simulink model "sf_bridge"  (Simulink 7.6)
settings: Solver=ode45  StartTime=0.0  StopTime=inf  RelTol=1e-3
libraries: sf_bidder x4, simulink x1
CloseFcn:
  | delete(findall(0, 'type', 'figure', 'tag', 'SF_BRIDGE'));
settings Model: Creator=The MathWorks Inc.  CovMetricSettings=dcmtr  ExtModeAutoUpdateStatusClock=off
settings DataIOCC: SignalLoggingName=sigsOut
settings OptimizationCC: InitFltsAndDblsToZero=on
settings DebuggingCC: SaveWithParameterizedLinksMsg=none  CheckExecutionContextPreStartOutputMsg=on  CheckExecutionContextRuntimeOutputMsg=on  SignalResolutionControl=TryResolveAllWithWarning  SolverPrmCheckMsg=none  MultiTaskDSMMsg=warning  MultiTaskCondExecSysMsg=none  StrictBusMsg=None
settings HardwareCC: TargetUnknown=on
settings SFSimCC: SFSimOverflowDetection=off  SimParseCustomCode=off
settings RTWCC: IncludeERTFirstTime=on
settings GRTTargetCC: TargetFcnLib=ansi_tfl_tmw.mat

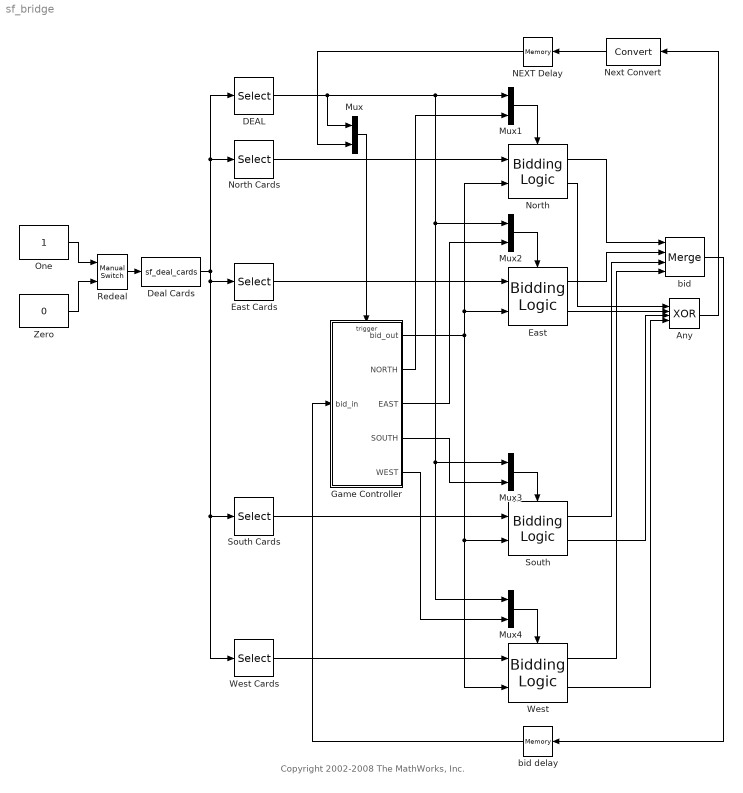
== system sf_bridge ==
  note: Copyright 2002-2008 The MathWorks, Inc.
  Any : Logic  Operator=XOR  Inputs=4  AllPortsSameDT=off
  DEAL : Selector  InputPortWidth=53  IndexOptions=Index vector (dialog)  Indices=[1]  OutputSizes=1
  Deal Cards : MATLABFcn  MATLABFcn=sf_deal_cards  OutputDimensions=53
  East : sf_bidder/Bidding Logic  SystemSampleTime=-1
  East Cards : Selector  InputPortWidth=53  IndexOptions=Index vector (dialog)  Indices=[15:27]  OutputSizes=1
  Game Controller : Stateflow chart  TreatAsAtomicUnit=on
  Mux{,1..4} (5 alike) : Mux  Inputs=2
  NEXT Delay : Memory
  Next Convert : DataTypeConversion  SaturateOnIntegerOverflow=on  RndMeth=Zero
  North : sf_bidder/Bidding Logic  SystemSampleTime=-1
  North Cards : Selector  InputPortWidth=53  IndexOptions=Index vector (dialog)  Indices=[2:14]  OutputSizes=1
  One : Constant
  Redeal : simulink/Signal Routing/Manual Switch  SystemSampleTime=-1  sw=0  action=0  varsize=off
  South : sf_bidder/Bidding Logic  SystemSampleTime=-1
  South Cards : Selector  InputPortWidth=53  IndexOptions=Index vector (dialog)  Indices=[28:40]  OutputSizes=1
  West : sf_bidder/Bidding Logic  SystemSampleTime=-1
  West Cards : Selector  InputPortWidth=53  IndexOptions=Index vector (dialog)  Indices=[41:53]  OutputSizes=1
  Zero : Constant  Value=0
  bid : Merge  Inputs=4
  bid delay : Memory
  wires:
  Deal Cards/1 -> DEAL/1, North Cards/1, West Cards/1, South Cards/1, East Cards/1
  DEAL/1 -> Mux/1, Mux1/1, Mux2/1, Mux4/1, Mux3/1
  bid/1 -> bid delay/1
  Any/1 -> Next Convert/1
  North Cards/1 -> North/1
  East Cards/1 -> East/1
  South Cards/1 -> South/1
  West Cards/1 -> West/1
  Game Controller/1(bid_out) -> South/2, West/2, North/2, East/2
  North/1 -> bid/1
  East/1 -> bid/2
  South/1 -> bid/3
  West/1 -> bid/4
  bid delay/1 -> Game Controller/1(bid_in)
  NEXT Delay/1 -> Mux/2
  Mux/1 -> Game Controller/Trigger
  North/2 -> Any/1
  West/2 -> Any/4
  East/2 -> Any/2
  South/2 -> Any/3
  Next Convert/1 -> NEXT Delay/1
  Mux1/1 -> North/Trigger
  Mux2/1 -> East/Trigger
  Mux3/1 -> South/Trigger
  Mux4/1 -> West/Trigger
  Game Controller/2(NORTH) -> Mux1/2
  Game Controller/3(EAST) -> Mux2/2
  Game Controller/4(SOUTH) -> Mux3/2
  Game Controller/5(WEST) -> Mux4/2
  Redeal/1 -> Deal Cards/1
  One/1 -> Redeal/1
  Zero/1 -> Redeal/2

== stateflow chart Game Controller ==
  state Bidder [parallel]
    settings: executionOrder=1
    state North
      NORTH;
    state East
      EAST;
    state South
      SOUTH;
    state West
      WEST;
    state Done
    Bidder -> (junction 21) [order 1] : BID
        | {process_bid();}
    Bidder.South -> Bidder.West : NEXT_BID
    Bidder.West -> Bidder.North : NEXT_BID
    Bidder.North -> Bidder.East : NEXT_BID
    Bidder.East -> Bidder.South : NEXT_BID
    (default) -> Done
    Done -> Bidder.North [order 2] : N_DEAL
    Done -> Bidder.East [order 1] : E_DEAL
    Done -> Bidder.South [order 4] : S_DEAL
    Done -> Bidder.West [order 3] : W_DEAL
    Bidder -> (junction 15) [order 3] : DEAL
        | {pass_count = 0;
        | bid_out = 0;}
    Bidder -> Done [order 2] : ALL_PASS
        | {ml.sf_bridge_state('all_pass');}
  state process_bid() [function]
    (junction 20) -> (junction 17) [order 1] : [bid_out]
        | {ALL_PASS;}
    (junction 20) -> (junction 24) [order 2] : {NEXT_BID;}
    (junction 19) -> (junction 23) [order 3] : {NEXT_BID;}
    (junction 16) -> (junction 19) [order 2] : {pass_count++;}
    (junction 16) -> (junction 18) [order 1] : [bid_in]
        | {pass_count = 0;
        | bid_out = bid_in;
        | NEXT_BID;}
    (junction 19) -> (junction 22) [order 1] : [pass_count == 4]
        | {ALL_PASS;}
    (default) -> (junction 16) : {ml.sf_bridge_state('bid', bid_in);}
    (junction 19) -> (junction 20) [order 2] : [pass_count == 3]
  state Dealer [parallel]
    settings: executionOrder=2
    state North
      ml.sf_bridge_state('deal', 'North');
      N_DEAL;
    state West
      ml.sf_bridge_state('deal', 'West');
      W_DEAL;
    state East
      ml.sf_bridge_state('deal', 'East');
      E_DEAL;
    state South
      ml.sf_bridge_state('deal', 'South');
      S_DEAL;
    Dealer.West -> Dealer.North : DEAL
    (default) -> Dealer.North
    Dealer.South -> Dealer.West : DEAL
    Dealer.North -> Dealer.East : DEAL
    Dealer.East -> Dealer.South : DEAL
  data: bid_in input uint8 size=1; bid_out output uint8 size=1; pass_count local uint8 size=1
  events: DEAL input EITHER_EDGE_EVENT; NORTH output EITHER_EDGE_EVENT; EAST output EITHER_EDGE_EVENT; SOUTH output EITHER_EDGE_EVENT; WEST output EITHER_EDGE_EVENT; BID input EITHER_EDGE_EVENT; E_DEAL local EITHER_EDGE_EVENT; NEXT_BID local EITHER_EDGE_EVENT; N_DEAL local EITHER_EDGE_EVENT; S_DEAL local EITHER_EDGE_EVENT; W_DEAL local EITHER_EDGE_EVENT; ALL_PASS local EITHER_EDGE_EVENT
